simulink model "TaskSpaceControl"  (Simulink 10.2)
settings: Solver=ode3  StartTime=0.0  StopTime=15  FixedStep=0.05  RelTol=1e-3  EnableMultiTasking=on
values from neighbouring files (symbols this model uses):
  q0 = [-pi/2;0]    [SetupConstants.m]
undefined symbols (not defined in the file or in its folder): Kpo, Kvomega, o_desired
libraries: vrlib x1, simulink x1
settings Model: Creator=Tim Salcudean  LastModifiedBy=jasper
settings SolverCC: ZeroCrossControl=DisableAll
settings DataIOCC: ExternalInput=[q0, u]  LimitDataPoints=on
settings OptimizationCC: ExpressionDepthLimit=2147483647  InitFltsAndDblsToZero=on
settings DebuggingCC: SaveWithParameterizedLinksMsg=none  SignalResolutionControl=TryResolveAllWithWarning  MaxConsecutiveZCsMsg=warning  MultiTaskDSMMsg=warning  MultiTaskCondExecSysMsg=none  StateNameClashWarn=warning
settings SFSimCC: SimParseCustomCode=off
settings GRTTargetCC: TargetFcnLib=ansi_tfl_tmw.mat

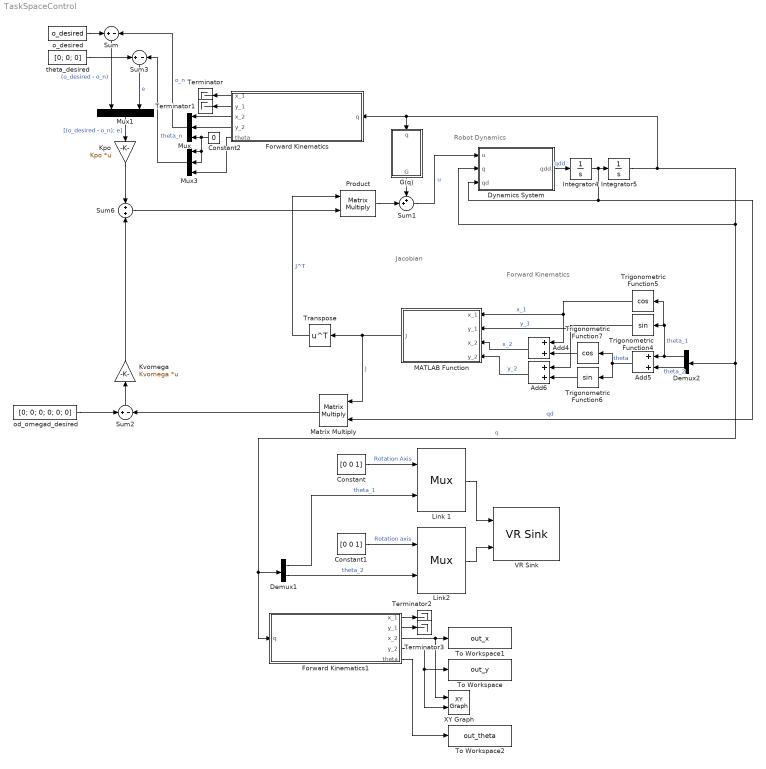
== system TaskSpaceControl ==
  note: Forward Kinematics
  note: Jacobian
  note: Robot Dynamics
  Add4 : Sum
  Add5 : Sum
  Add6 : Sum
  Constant : Constant  Value=[0 0 1]
  Constant1 : Constant  Value=[0 0 1]
  Constant2 : Constant  Value=0
  Demux1 : Demux  Outputs=2
  Demux2 : Demux  Outputs=2
  Dynamics System : MATLAB Function  TreatAsAtomicUnit=on
  Forward Kinematics : Subsystem
  Forward Kinematics1 : Subsystem
  G(q) : MATLAB Function  TreatAsAtomicUnit=on
  Integrator4 : Integrator  InitialCondition=[0;0]
  Integrator5 : Integrator  InitialCondition=q0
  Kpo : Gain  Gain=Kpo  Multiplication=Matrix(K*u)
  Kvomega : Gain  Gain=Kvomega  Multiplication=Matrix(K*u)
  Link 1 : Mux  Inputs=2
      settings: DisplayOption=signals
  Link2 : Mux  Inputs=2
      settings: DisplayOption=signals
  MATLAB Function : MATLAB Function  TreatAsAtomicUnit=on
  Matrix Multiply : Product  Multiplication=Matrix(*)
  Mux : Mux  Inputs=3
  Mux1 : Mux  Inputs=2
  Mux3 : Mux  Inputs=3
  Product : Product  Multiplication=Matrix(*)
  Sum : Sum  Inputs=+|-
  Sum1 : Sum  Inputs=++|
  Sum2 : Sum  Inputs=+|-
  Sum3 : Sum  Inputs=+|-
  Sum6 : Sum  Inputs=+|+
  Terminator{,1..3} (4 alike) : Terminator
  To Workspace : ToWorkspace  VariableName=out_y  SaveFormat=Timeseries  SampleTime=-1
  To Workspace1 : ToWorkspace  VariableName=out_x  SaveFormat=Timeseries  SampleTime=-1
  To Workspace2 : ToWorkspace  VariableName=out_theta  SaveFormat=Timeseries  SampleTime=-1
  Transpose : Math  Operator=transpose  SaturateOnIntegerOverflow=on
  Trigonometric Function4 : Trigonometry
  Trigonometric Function5 : Trigonometry  Operator=cos
  Trigonometric Function6 : Trigonometry
  Trigonometric Function7 : Trigonometry  Operator=cos
  VR Sink : vrlib/VR Sink  InstantiateOnLoad=on  SampleTime=-1  ViewEnable=on  RemoteChange=off  RemoteView=off  FieldsWritten=Link1.rotation.4.1.double#Link2.rotation.4.1.double  WorldFileName=HalfScara.WRL  AutoView=off  VideoDimensions=[]  AllowVariableSize=off
  XY Graph : simulink/Sinks/XY Graph  xmin=-2  xmax=2  ymin=-2  ymax=2  st=-1
  o_desired : Constant  Value=o_desired  VectorParams1D=off
  od_omegad_desired : Constant  Value=[0; 0; 0; 0; 0; 0]  VectorParams1D=off
  theta_desired : Constant  Value=[0; 0; 0]  VectorParams1D=off
  wires:
  Constant/1 -> Link 1/1  "Rotation Axis"
  Constant1/1 -> Link2/1  "Rotation axis"
  Link 1/1 -> VR Sink/1
  Link2/1 -> VR Sink/2
  Sum2/1 -> Kvomega/1
  G(q)/1(G) -> Sum1/1
  Sum1/1 -> Dynamics System/1(u)  "u"
  Integrator4/1 -> Matrix Multiply/2, Dynamics System/3(qd), Integrator5/1  "qd"
  Dynamics System/1(qdd) -> Integrator4/1  "qdd"
  Mux/1 -> Sum/2  "o_n"
  MATLAB Function/1(J) -> Transpose/1, Matrix Multiply/1  "J"
  od_omegad_desired/1 -> Sum2/1
  Matrix Multiply/1 -> Sum2/2
  Product/1 -> Sum1/2
  Kvomega/1 -> Sum6/2
  Add4/1 -> MATLAB Function/3(x_2)  "x_2"
  Demux2/1 -> Trigonometric Function5/1, Trigonometric Function4/1, Add5/1  "theta_1"
  Add6/1 -> MATLAB Function/4(y_2)  "y_2"
  Trigonometric Function4/1 -> Add6/1, MATLAB Function/2(y_1)  "y_1"
  Trigonometric Function5/1 -> Add4/1, MATLAB Function/1(x_1)  "x_1"
  Demux2/2 -> Add5/2  "theta_2"
  Trigonometric Function6/1 -> Add6/2
  Add5/1 -> Trigonometric Function6/1, Trigonometric Function7/1  "theta"
  Trigonometric Function7/1 -> Add4/2
  Forward Kinematics/3(x_2) -> Mux/1
  Forward Kinematics/4(y_2) -> Mux/2
  Forward Kinematics/1(x_1) -> Terminator/1
  Forward Kinematics/2(y_1) -> Terminator1/1
  o_desired/1 -> Sum/1
  theta_desired/1 -> Sum3/1
  Sum3/1 -> Mux1/2  "e"
  Sum/1 -> Mux1/1  "(o_desired - o_n)"
  Kpo/1 -> Sum6/1
  Mux1/1 -> Kpo/1  "[(o_desired - o_n); e]"
  Demux1/2 -> Link2/2  "theta_2"
  Demux1/1 -> Link 1/2  "theta_1"
  Integrator5/1 -> Demux1/1, Forward Kinematics1/1(q), Demux2/1, Dynamics System/2(q), G(q)/1(q), Forward Kinematics/1(q)  "q"
  Forward Kinematics1/3(x_2) -> XY Graph/1, To Workspace1/1
  Forward Kinematics1/4(y_2) -> XY Graph/2, To Workspace/1
  Forward Kinematics1/5(theta) -> To Workspace2/1
  Forward Kinematics1/1(x_1) -> Terminator2/1
  Forward Kinematics1/2(y_1) -> Terminator3/1
  Constant2/1 -> Mux3/2, Mux3/1, Mux/3
  Forward Kinematics/5(theta) -> Mux3/3
  Mux3/1 -> Sum3/2  "theta_n"
  Transpose/1 -> Product/1  "J^T"
  Sum6/1 -> Product/2

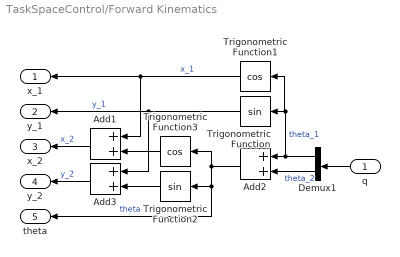
== system TaskSpaceControl/Forward Kinematics ==
  q : Inport
  Add1 : Sum
  Add2 : Sum
  Add3 : Sum
  Demux1 : Demux  Outputs=2
  Trigonometric Function : Trigonometry
  Trigonometric Function1 : Trigonometry  Operator=cos
  Trigonometric Function2 : Trigonometry
  Trigonometric Function3 : Trigonometry  Operator=cos
  x_1 : Outport
  y_1 : Outport  Port=2
  x_2 : Outport  Port=3
  y_2 : Outport  Port=4
  theta : Outport  Port=5
  wires:
  Trigonometric Function2/1 -> Add3/2
  q/1 -> Demux1/1
  Add3/1 -> y_2/1  "y_2"
  Demux1/2 -> Add2/2  "theta_2"
  Add1/1 -> x_2/1  "x_2"
  Add2/1 -> theta/1, Trigonometric Function2/1, Trigonometric Function3/1  "theta"
  Trigonometric Function/1 -> Add3/1, y_1/1  "y_1"
  Trigonometric Function3/1 -> Add1/2
  Demux1/1 -> Trigonometric Function1/1, Trigonometric Function/1, Add2/1  "theta_1"
  Trigonometric Function1/1 -> Add1/1, x_1/1  "x_1"

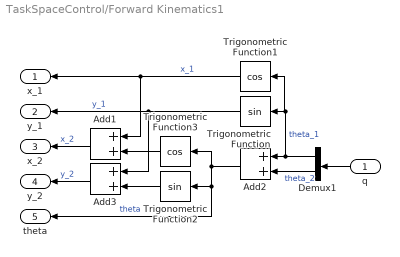
== system TaskSpaceControl/Forward Kinematics1 ==
  q : Inport
  Add1 : Sum
  Add2 : Sum
  Add3 : Sum
  Demux1 : Demux  Outputs=2
  Trigonometric Function : Trigonometry
  Trigonometric Function1 : Trigonometry  Operator=cos
  Trigonometric Function2 : Trigonometry
  Trigonometric Function3 : Trigonometry  Operator=cos
  x_1 : Outport
  y_1 : Outport  Port=2
  x_2 : Outport  Port=3
  y_2 : Outport  Port=4
  theta : Outport  Port=5
  wires:
  Trigonometric Function2/1 -> Add3/2
  q/1 -> Demux1/1
  Add3/1 -> y_2/1  "y_2"
  Demux1/2 -> Add2/2  "theta_2"
  Add1/1 -> x_2/1  "x_2"
  Add2/1 -> theta/1, Trigonometric Function2/1, Trigonometric Function3/1  "theta"
  Trigonometric Function/1 -> Add3/1, y_1/1  "y_1"
  Trigonometric Function3/1 -> Add1/2
  Demux1/1 -> Trigonometric Function1/1, Trigonometric Function/1, Add2/1  "theta_1"
  Trigonometric Function1/1 -> Add1/1, x_1/1  "x_1"

== matlab function G(q) ==
  data: q input double; G output double
function G = G(q)

g=9.81;
theta1=q(1);
theta2=q(2);
G=[2*g*cos(theta1)+g*cos(theta1+theta2); g*cos(theta1+theta2)];

== matlab function MATLAB Function ==
  data: x_1 input double; J output double; y_1 input double; x_2 input double; y_2 input double
function J = jacobian(x_1, y_1, x_2, y_2)

J = robot_jacobian(x_1, y_1, x_2, y_2);

== matlab function Dynamics System ==
  data: u input double; q input double; qdd output double; qd input double
function qdd  = dynamics(u, q, qd)

g=9.81;
theta1=q(1);
theta2=q(2);
theta1d=qd(1);
theta2d=qd(2);
D=[3+2*cos(theta2) 1+cos(theta2); 1+cos(theta2) 1];
C=[-2*sin(theta2)*theta2d -sin(theta2)*theta2d; sin(theta2)*theta1d 0];
G=[2*g*cos(theta1)+g*cos(theta1+theta2); g*cos(theta1+theta2)];

qdd=inv(D)*(u-G-C*qd);
